simulink model "TrayectoriaStateFlow"  (R2023b)
settings: Solver=FixedStepAuto  StartTime=0.0  StopTime=65  RelTol=1e-3  EnableMultiTasking=on
model workspace (MAT data in the model file):
  d = 0.24
settings Model: PacingRate=1.500000  ExtModeTrigDuration=2  Creator=manu_  LastModifiedBy=manu_
settings OptimizationCC: EnhancedBackFolding=on  PassReuseOutputArgsAs=Individual arguments  ZeroExternalMemoryAtStartup=off  ZeroInternalMemoryAtStartup=off  MaxStackSize=64  OptimizeBlockOrder=speed  DifferentSizesBufferReuse=on  EfficientTunableParamExpr=on
settings DebuggingCC: ParameterTunabilityLossMsg=error
settings HardwareCC: ProdBitPerInt=16  ProdBitPerPointer=16  ProdBitPerSizeT=16  ProdBitPerPtrDiffT=16  ProdLargestAtomicFloat=None  ProdWordSize=8  ProdHWDeviceType=Atmel->AVR  UseEmbeddedCoderFeatures=off  UseSimulinkCoderFeatures=off
settings SFSimCC: MATLABDynamicMemAlloc=off
settings RTWCC: Description=Embedded Coder  SystemTargetFile=ert.tlc  HardwareBoard=Arduino Mega 2560  TemplateMakefile=ert_default_tmf  Toolchain=Arduino AVR  BuildConfiguration=Faster Runs
settings CodeAppCC: ForceParamTrailComments=on  IgnoreCustomStorageClasses=off  OperatorAnnotations=on  SimulinkDataObjDesc=on  SFDataObjDesc=on  InsertBlockDesc=on
settings ERTTargetCC: SupportContinuousTime=on  SupportNonInlinedSFcns=on  SupportVariableSizeSignals=on  ExtModeTransport=3  ExtModeStaticAlloc=on  ExtModeAutomaticAllocSize=off  ExtModeStaticAllocSize=2048  ExtModeMexFile=ext_xcp  ExtModeIntrfLevel=Level2 - Open

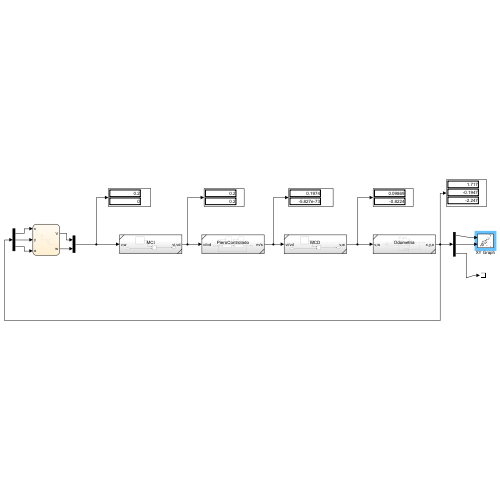
[thumbnail: Simulink's stored preview of the top-level diagram]
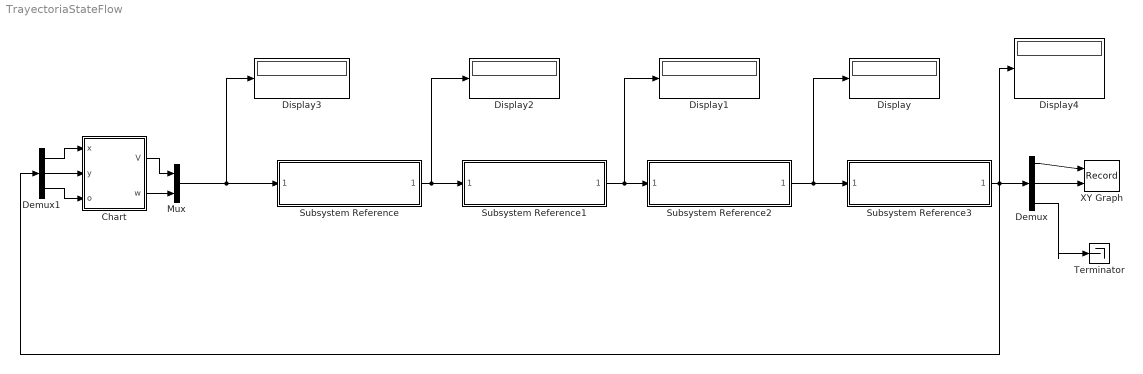
== system TrayectoriaStateFlow ==
  Chart : Stateflow chart  TreatAsAtomicUnit=on
      settings: PortSchema="{\"entries\":[{\"content\":{\"sides\":[{\"content\":{\"connectorIds\":[\"In1\",\"In3\",\"In2\"]},\"type\":\"ConnectorPlacement.EquallySpacedRectSide\",\"uuid\":\"907b1d5e-09da-4342-ad4d-4adfc9d3eca5\"},{\"content\":{\"connectorIds\":[\"Out1\",\"Out2\"],\"side\":\"RIGHT\"},\"type\":\"ConnectorPlacement.EquallySpacedRectSide\",\"uuid\":\"a2530904-a383-4ac0-a414-663b94632794\"},{\"content\":{\"side\":\"TOP\"},\"type\":\"ConnectorPlacement.EquallySpacedRectSide\",\"uuid\":\"49c3c5b9-d2e2-4189-8dc1-6ae705df0e89\"}]},\"type\":\"ConnectorPlacement.EquallySpacedConnector\",\"uuid\":\"371d9772-85a1-4e1f-9fbe-365c52e303c6\"}],\"packageUris\":[\"http://schema.mathworks.com/mf0/Connector/R2020b\"],\"version\":\"1.0\"}"
  Demux : Demux  Outputs=3
  Demux1 : Demux  Outputs=3
  Display{,1..4} (5 alike) : Display
  Mux : Mux  Inputs=2
  Subsystem Reference : Subsystem  ReferencedSubsystem=MCI
  Subsystem Reference1 : Subsystem  ReferencedSubsystem=PieroControlado
  Subsystem Reference2 : Subsystem  ReferencedSubsystem=MCD
  Subsystem Reference3 : Subsystem  ReferencedSubsystem=Odometria
  Terminator : Terminator
  XY Graph : Record  FileSettingsInternal="{\"entries\":[{\"content\":{\"excelSettings\":{\"content\":{},\"type\":\"Streamout.ExcelSettings\"}},\"type\":\"Streamout.FileSettingStorage\",\"uuid\":\"\"}],\"packageUris\":[\"http:\\/\\/schema.mathworks.com\\/mf0\\/streamout_blocks\\/R2020a\"],\"version\":\"1.0\"}"  Layout=[1 1]  SignalsInternal="{\"entries\":[{\"content\":{\"signals\":[{\"content\":{\"blockPath\":[],\"dimensions\":[1],\"domain\":\"\",\"lineColor\":\"#a2142f\",\"plots\":[ 1 ],\"port\":1,\"sid\":[\"\"],\"signalID\":1,\"signalName\":\"Demux:1\"},\"type\":\"RecordBlkView.Signal\",\"uuid\":\"\"},{\"content\":{\"blockPath\":[],\"dimensions\":[1],\"domain\":\"\",\"lineColor\":\"#139fff\",\"plots\":[ 1 ],\"port\":2,\"sid\":[\"\"],\"signalID\":2,\"signalName\":\"Demux:2\"},\"type\":\"RecordBlkView.Signal\",\"uuid\":\"\"}]},\"type\":\"RecordBlkView.InputSignals\",\"uuid\":\"\"}],\"packageUris\":[\"http:\\/\\/schema.mathworks.com\\/mf0\\/streamout_blocks\\/R2020a\"],\"version\":\"1.0\"}"  VisualizationBindings="{\"xyplotplugin\":{\"info\":[{\"series\":[{\"bindingParametersList\":[{\"parameter\":\"X-Axis\",\"signalID\":1,\"signalName\":\"Demux:1\"},{\"parameter\":\"Y-Axis\",\"signalID\":2,\"signalName\":\"Demux:2\"}],\"seriesID\":0}],\"subplotID\":1}]}}"  CompatibilityTag=XY
  wires:
  Subsystem Reference/1 -> Display2/1, Subsystem Reference1/1
  Subsystem Reference2/1 -> Display/1, Subsystem Reference3/1
  Subsystem Reference1/1 -> Display1/1, Subsystem Reference2/1
  Subsystem Reference3/1 -> Demux1/1, Display4/1, Demux/1
  Demux/2 -> XY Graph/2
  Demux/1 -> XY Graph/1
  Demux/3 -> Terminator/1
  Chart/1(V) -> Mux/1
  Chart/2(w) -> Mux/2
  Mux/1 -> Display3/1, Subsystem Reference/1
  Demux1/1 -> Chart/1(x)
  Demux1/2 -> Chart/3(y)
  Demux1/3 -> Chart/2(o)

== stateflow chart TrayectoriaStateFlow/Chart ==
  state Inicio
    entry:
    V=0;
    w=0;
  state Recto1
    entry:
    V=0.2;
    w=0;
  state GiroDch1
    entry:
    V=0;
    w=-pi/4;
  state Recto2
    entry:
    V=0.2;
    w=0;
  state GiroDch2
    entry:
    V=0;
    w=-pi/4;
  state GiroIzq1
    entry:
    V=0;
    w=pi/4
  state Recto3
    entry:
    V=0.2;
    w=0;
  state Recto4
    entry:
    V=0.2;
    w=0;
  state GiroIzq2
    entry:
    V=0;
    w=pi/4;
  state Recto5
    entry:
    V=0.2;
    w=0;
  state GiroDch3
    entry:
    V=0;
    w=-pi/4;
  state Recto6
    entry:
    V=0.2
    w=0;
  state Final
    entry:
    V=0;
    w=0;
  (default) -> Inicio
  Inicio -> Recto1 : after(1,sec)
  Recto1 -> GiroDch1 : [x>1.6]
  GiroDch1 -> Recto2 : [o<-pi/2]
  Recto2 -> GiroIzq1 : [y<-1.6]
  GiroIzq1 -> Recto3 : [o<0]
  Recto3 -> GiroDch2 : [x>2.6]
  GiroDch2 -> Recto4 : [o<=-pi/2]
  Recto4 -> GiroIzq2 : [y>=4.4]
  GiroIzq2 -> Recto5 : [o>=0]
  Recto5 -> GiroDch3 : [x>=3.2]
  GiroDch3 -> Recto6 : [o<=-pi/2]
  Recto6 -> Final : [y>=5]
  data: x input; o input; V output double size=1; w output double size=1; y input
